simulink model "dc3_szabalyzo"  (R2013a)
settings: Solver=VariableStepDiscrete  StartTime=0.0  StopTime=20  RelTol=1e-3
undefined symbols (not defined in the file or in its folder): j
settings Model: Creator=balazs.varga  LastModifiedBy=balazs.varga

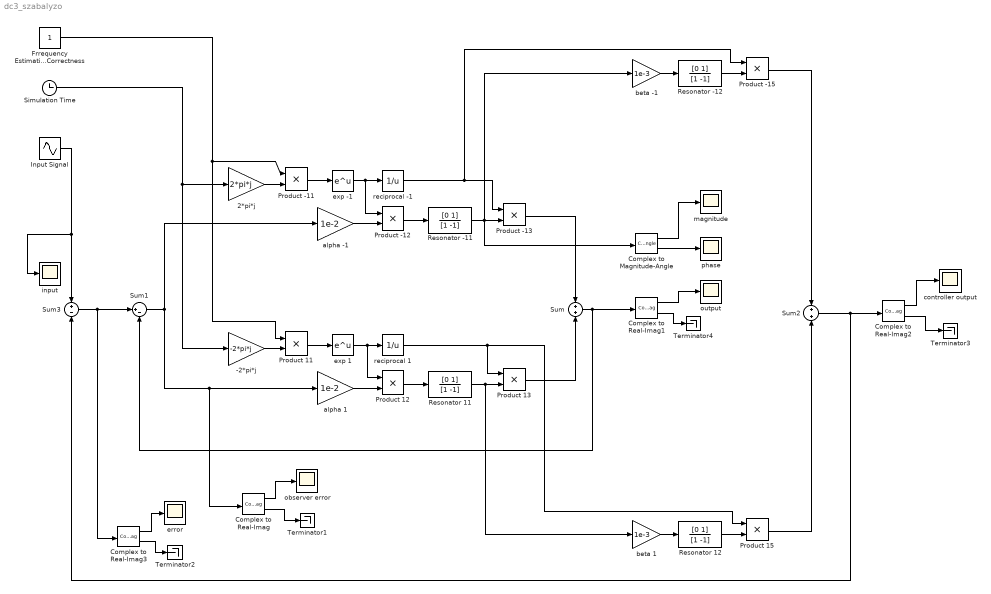
== system dc3_szabalyzo ==
  -2*pi*j : Gain  Gain=-2*pi*j  SampleTime=1e-3
  2*pi*j : Gain  Gain=2*pi*j  SampleTime=1e-3
  Complex to Magnitude-Angle : ComplexToMagnitudeAngle  SampleTime=1e-3
  Complex to Real-Imag{,1..3} (4 alike) : ComplexToRealImag  SampleTime=1e-3
  Frrequency Estimation Correctness : Constant
  Input Signal : Sin  Amplitude=1.5  Frequency=2*pi  Phase=1  SampleTime=0
  Product -{11..13,15} (4 alike) : Product  SampleTime=1e-3
  Product {11..13,15} (4 alike) : Product  SampleTime=1e-3
  Resonator -11 : DiscreteFilter  Numerator=[0 1]  Denominator=[1 -1]  SampleTime=1e-3
  Resonator -12 : DiscreteFilter  Numerator=[0 1]  Denominator=[1 -1]  SampleTime=1e-3
  Resonator 11 : DiscreteFilter  Numerator=[0 1]  Denominator=[1 -1]  SampleTime=1e-3
  Resonator 12 : DiscreteFilter  Numerator=[0 1]  Denominator=[1 -1]  SampleTime=1e-3
  Simulation Time : Clock
  Sum : Sum  Inputs=+|+  SampleTime=1e-3
  Sum1 : Sum  Inputs=|+-  SampleTime=1e-3
  Sum2 : Sum  Inputs=+|+  SampleTime=1e-3
  Sum3 : Sum  Inputs=+|-  SampleTime=1e-3
  Terminator{1..4} (4 alike) : Terminator
  alpha -1 : Gain  Gain=1e-2  SampleTime=1e-3
  alpha 1 : Gain  Gain=1e-2  SampleTime=1e-3
  beta -1 : Gain  Gain=1e-3  SampleTime=1e-3
  beta 1 : Gain  Gain=1e-3  SampleTime=1e-3
  "controller output " : Scope
      settings: YMin=-7  YMax=7  SaveName=ScopeData5
  error : Scope
      settings: YMin=-1.5  YMax=1.5  SaveName=ScopeData6
  exp -1 : Math  SampleTime=1e-3  SaturateOnIntegerOverflow=on
  exp 1 : Math  SampleTime=1e-3  SaturateOnIntegerOverflow=on
  input : Scope
      settings: SaveName=ScopeData2
  magnitude : Scope
      settings: SaveName=ScopeData3
  observer error : Scope
  output : Scope
  phase : Scope
      settings: SaveName=ScopeData4
  reciprocal -1 : Math  Operator=reciprocal  SampleTime=1e-3  SaturateOnIntegerOverflow=on
  reciprocal 1 : Math  Operator=reciprocal  SampleTime=1e-3  SaturateOnIntegerOverflow=on
  wires:
  Product -12/1 -> Resonator -11/1
  Product 12/1 -> Resonator 11/1
  Product -11/1 -> exp -1/1
  Product 11/1 -> exp 1/1
  Simulation Time/1 -> -2*pi*j/1, 2*pi*j/1
  exp -1/1 -> reciprocal -1/1, Product -12/1
  Resonator -11/1 -> beta -1/1, Complex to Magnitude-Angle/1, Product -13/2
  exp 1/1 -> reciprocal 1/1, Product 12/1
  Resonator 11/1 -> beta 1/1, Product 13/2
  Product -13/1 -> Sum/1
  Product 13/1 -> Sum/2
  Sum/1 -> Complex to Real-Imag1/1, Sum1/2
  Sum1/1 -> Complex to Real-Imag/1, alpha 1/1, alpha -1/1
  Complex to Real-Imag/1 -> observer error/1
  Complex to Real-Imag1/1 -> output/1
  Complex to Magnitude-Angle/1 -> magnitude/1
  Complex to Magnitude-Angle/2 -> phase/1
  Frrequency Estimation Correctness/1 -> Product 11/1, Product -11/1
  beta -1/1 -> Resonator -12/1
  Resonator -12/1 -> Product -15/2
  beta 1/1 -> Resonator 12/1
  Resonator 12/1 -> Product 15/2
  Product -15/1 -> Sum2/1
  Product 15/1 -> Sum2/2
  Complex to Real-Imag2/1 -> "controller output "/1
  reciprocal 1/1 -> Product 15/1, Product 13/1
  reciprocal -1/1 -> Product -15/1, Product -13/1
  Input Signal/1 -> Sum3/1, input/1
  Sum3/1 -> Sum1/1, Complex to Real-Imag3/1
  Sum2/1 -> Complex to Real-Imag2/1, Sum3/2
  Complex to Real-Imag3/1 -> error/1
  Complex to Real-Imag/2 -> Terminator1/1
  Complex to Real-Imag3/2 -> Terminator2/1
  Complex to Real-Imag2/2 -> Terminator3/1
  Complex to Real-Imag1/2 -> Terminator4/1
  -2*pi*j/1 -> Product 11/2
  2*pi*j/1 -> Product -11/2
  alpha 1/1 -> Product 12/2
  alpha -1/1 -> Product -12/2
